simulink model "eovsa_corr_300mhz"  (R2012b)
settings: Solver=VariableStepDiscrete  SolverMode=SingleTasking  StartTime=0.0  StopTime=5000  RelTol=1e-3
undefined symbols (not defined in the file or in its folder): A, B, gcbh, PCIN, sfp, xlBlockLoadCallback, xlipgetpartsetting
libraries: xbsIndex_r4 x5996, casper_library_misc x52, simulink x33, dspsigops x24, xps_library x15, casper_library_delays x2
(part 5 of 65)

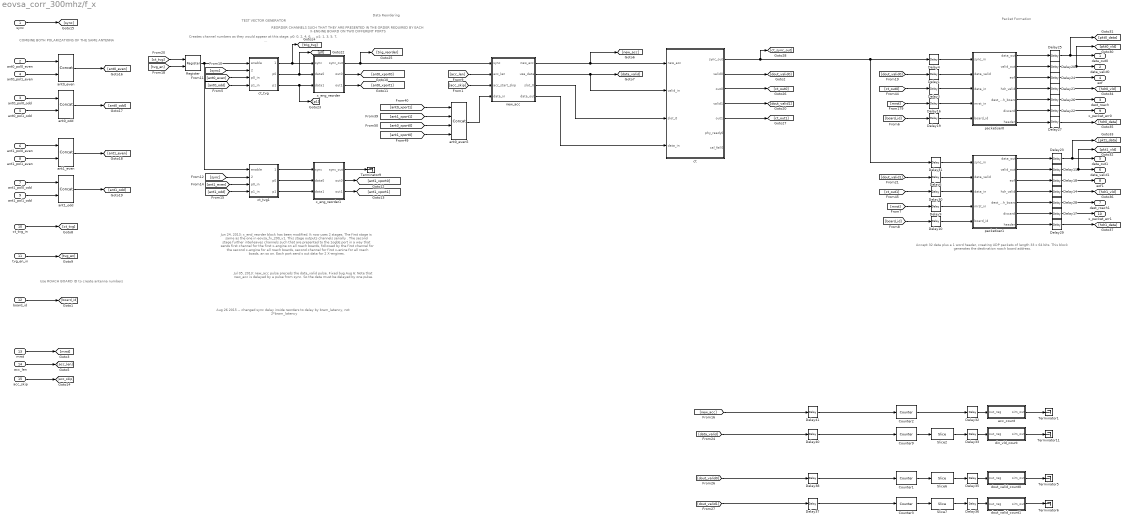
== system eovsa_corr_300mhz/f_x ==
  note: Aug 26 2015 -- changed sync delay inside reorders to delay by bram_latency, not 2*bram_latency
  note: Accept 32 data plus a 1 word header,
      | creating UDP packets of length 33 x 64 bits.
      | This block generates the destination roach board address.
  note: Packet Formation
  note: Data Reordering
  note: COMBINE BOTH POLARIZATIONS
      | OF THE SAME ANTENNA
  note: REORDER CHANNELS SUCH THAT
      | THEY ARE PRESENTED IN THE ORDER
      | REQUIRED BY EACH X-ENGINE BOARD
      | ON TWO DIFFERENT PORTS
  note: TEST VECTOR
      | GENERATOR
  note: Creates channel numbers as they
      | would appear at this stage.
      | p0: 0, 2, 4, 6, ...
      | p1: 1, 3, 5, 7, ...
  note: Jun 24, 2013: x_end_reorder block has been modified.
      | It now uses 2 stages. The first stage is same as the one in eovsa_fx_200_v1.
      | This stage outputs channels serially .
      | The second stage further interleaves channels such that are presented to the 1ogbE port in a way that sends first channel for the first x-engine on all roach boards, followed by
      | the first channel for the second x-engine for all roach boards, second channel for first x-enine for all roach boads, an so on. Each port send s out data for 2 X-engines.
  note: Use ROACH BOARD ID to create antenna numbers
  note: Jul 05, 2013: new_acc  pulse preceds the data_valid pulse. Fixed bug
      | Aug 6: Note that new_acc is delayed by a pulse from sync. So the data must be delayed by one pulse.
  sync : Inport
  ant0_pol0_even : Inport  Port=2
  ant0_pol0_odd : Inport  Port=3
  ant0_pol1_even : Inport  Port=4
  ant0_pol1_odd : Inport  Port=5
  ant1_pol0_even : Inport  Port=6
  ant1_pol0_odd : Inport  Port=7
  ant1_pol1_even : Inport  Port=8
  ant1_pol1_odd : Inport  Port=9
  ct_tvg_in : Inport  Port=10
  tvg_en_in : Inport  Port=11
  board_id : Inport  Port=12
  mrst : Inport  Port=13
  acc_len : Inport  Port=14
  acc_skip : Inport  Port=15
  Counter1 : xbsIndex_r4/Counter  cnt_type=Free Running  cnt_to=Inf  operation=Up  start_count=0  cnt_by_val=1  arith_type=Unsigned  n_bits=32+13  bin_pt=0  load_pin=off  rst=off  en=on  explicit_period=off  period=1  dbl_ovrd=off  use_behavioral_HDL=off  implementation=DSP48  block_type=counter
      settings: block_version=11.4
  Counter2 : xbsIndex_r4/Counter  cnt_type=Free Running  cnt_to=Inf  operation=Up  start_count=0  cnt_by_val=1  arith_type=Unsigned  n_bits=32  bin_pt=0  load_pin=off  rst=off  en=on  explicit_period=off  period=1  dbl_ovrd=off  use_behavioral_HDL=off  implementation=DSP48  block_type=counter
      settings: block_version=11.4
  Counter3 : xbsIndex_r4/Counter  cnt_type=Free Running  cnt_to=Inf  operation=Up  start_count=0  cnt_by_val=1  arith_type=Unsigned  n_bits=32+13  bin_pt=0  load_pin=off  rst=off  en=on  explicit_period=off  period=1  dbl_ovrd=off  use_behavioral_HDL=off  implementation=DSP48  block_type=counter
      settings: block_version=11.4
  Counter9 : xbsIndex_r4/Counter  cnt_type=Free Running  cnt_to=Inf  operation=Up  start_count=0  cnt_by_val=1  arith_type=Unsigned  n_bits=46  bin_pt=0  load_pin=off  rst=off  en=on  explicit_period=off  period=1  dbl_ovrd=off  use_behavioral_HDL=off  implementation=DSP48  block_type=counter
      settings: block_version=11.4
  Delay{1,3,6,30,32..33,35..38,40..41} (12 alike) : xbsIndex_r4/Delay  rst=off  infoeditControl=Selection of Reset will increase slice count due to use of real FFs and instead of SRLs  en=off  latency=1  dbl_ovrd=off  reg_retiming=off  block_type=delay
      settings: xl_area=[0, 0, 0, 0, 0, 0, 0]
  Delay{4,9..11,14,16..29,31} (20 alike) : xbsIndex_r4/Delay  rst=off  infoeditControl=Selection of Reset will increase slice count due to use of real FFs and instead of SRLs  en=off  latency=1  dbl_ovrd=off  reg_retiming=on  block_type=delay
      settings: xl_area=[0, 0, 0, 0, 0, 0, 0]
  Register : xbsIndex_r4/Register  init=0  rst=off  en=on  dbl_ovrd=off  block_type=register
      settings: block_version=11.4
  Slice2 : xbsIndex_r4/Slice  nbits=32  boolean_output=off  mode=Upper Bit Location + Width  bit1=0  base1=MSB of Input  bit0=32  base0=LSB of Input  dbl_ovrd=off  block_type=slice
  Slice6 : xbsIndex_r4/Slice  nbits=32  boolean_output=off  mode=Upper Bit Location + Width  bit1=0  base1=MSB of Input  bit0=32  base0=LSB of Input  dbl_ovrd=off  block_type=slice
  Slice7 : xbsIndex_r4/Slice  nbits=32  boolean_output=off  mode=Upper Bit Location + Width  bit1=0  base1=MSB of Input  bit0=32  base0=LSB of Input  dbl_ovrd=off  block_type=slice
  Terminator{1,5..6,9,11} (5 alike) : Terminator
  acc_count : Subsystem  Tag=xps:sw_reg  AncestorBlock=xps_library/software_register  mask(swreg){mode=one value, io_dir=To Processor, io_delay=0, sample_period=1, names=reg, bitwidths=32, arith_types=0, bin_pts=0, sim_port=on, show_format=off}
      mask prompts: io_dir "I/O direction"; io_delay "I/O delay"; sample_period "Sample period"; names "Name:"; bitwidths "Bitwidth:"; arith_types "Type (ufix=0, fix=1, bool=2):"; bin_pts "Binary pt:"; sim_port "Provide sim input/output?"; show_format "Print format string?"
      mask init:
      | swreg_init(gcb)
      settings: AttributesFormatString=1output
      mask TypeOptions mode: one value | fields of equal size | fields of arbitrary size
      mask Callback mode: swreg_cb(gcb);
      mask TypeOptions io_dir: To Processor | From Processor
      mask Callback io_dir:
      | mask_enables = get_param(gcb, 'MaskEnables');
      | mask_names = get_param(gcb, 'MaskNames');
      | if strcmp(get_param(gcb, 'io_dir'), 'To Processor'),
      |     mask_enables{ismember(mask_names, 'sample_period')} = 'off';
      | else
      |     mask_enables{ismember(mask_names, 'sample_period')} = 'on';
      | end
      | set_param(gcb, 'MaskEnables', mask_enables);
      mask Callback bitwidths:
      | swreg_maskcheck(gcb);
      | % blk = gcb;
      | % mode = get_param(blk, 'mode');
      | % current_widths = eval(get_param(blk, 'bitwidths'));
      | % if (strcmp(mode, 'one value') || strcmp(mode, 'fields of equal size')) && (length(current_widths) > 1),
      | %     error('Only one width may be specified for this mode.');
      | % elseif strcmp(mode, 'fields of arbitrary size')
      | %     current_names = textscan(strtrim(strrep(strrep(get_param(blk, 'names'), ']', ''), '[', '')), '%s');
      | %     current_names = current_names{1};
      | %     numios = length(current_names);
      | %     if length(current_widths) ~= numios,
      | %         error('%d field names specified, but %d widths?', numios, length(current_widths));
      | %     end
      | % end
      | % total_width = 0;
      | % for ctr = 1 : length(current_widths),
      | %     total_width = total_width + current_widths(ctr);
      | % end
      | % if total_width > 32,
      | %     error('Total width must be 32 or less, set to %d.', total_width);
      | % end
      mask Callback arith_types:
      | [numios, ~, ~, ~, current_types] = swreg_maskcheck(gcb);
      | % blk = gcb;
      | % mode = get_param(blk, 'mode');
      | % current_types = eval(get_param(blk, 'arith_types'));
      | % numios = length(current_types);
      | % if (strcmp(mode, 'one value') || strcmp(mode, 'fields of equal size')) && (length(current_types) > 1),
      | %     error('Only one type may be specified for this mode.');
      | % elseif strcmp(mode, 'fields of arbitrary size')
      | %     current_names = textscan(strtrim(strrep(strrep(get_param(blk, 'names'), ']', ''), '[', '')), '%s');
      | %     current_names = current_names{1};
      | %     numios = length(current_names);
      | %     if length(current_types) ~= numios,
      | %         error('%d field names specified, but %d types?', numios, length(current_types));
      | %     end
      | % end
      | problem = 0;
      | for ctr = 1 : numios,
      |     t = current_types(ctr);
      |     if (t < 0) || (t > 2),
      |         problem = t;
      |         ctr = numios + 1;
      |     end
      | end
      | if problem ~= 0,
      |     error('Type cannot be %i, must be 0, 1 or 2.', problem);
      | end
      mask Callback bin_pts:
      | swreg_maskcheck(gcb);
      | % blk = gcb;
      | % mode = get_param(blk, 'mode');
      | % current_bins = eval(get_param(blk, 'bin_pts'));
      | % if (strcmp(mode, 'one value') || strcmp(mode, 'fields of equal size')) && (length(current_bins) > 1),
      | %     error('Only one binary pt may be specified for this mode.');
      | % elseif strcmp(mode, 'fields of arbitrary size')
      | %     current_names = textscan(strtrim(strrep(strrep(get_param(blk, 'names'), ']', ''), '[', '')), '%s');
      | %     current_names = current_names{1};
      | %     numios = length(current_names);
      | %     if length(current_bins) ~= numios,
      | %         error('%d field names specified, but %d binary pts?', numios, length(current_bins));
      | %     end
      | % end
  ant0_even : xbsIndex_r4/Concat  num_inputs=2  dbl_ovrd=off  block_type=concat
  ant0_even5 : xbsIndex_r4/Concat  num_inputs=4  dbl_ovrd=off  block_type=concat
  ant0_odd : xbsIndex_r4/Concat  num_inputs=2  dbl_ovrd=off  block_type=concat
  ant1_even : xbsIndex_r4/Concat  num_inputs=2  dbl_ovrd=off  block_type=concat
  ant1_odd : xbsIndex_r4/Concat  num_inputs=2  dbl_ovrd=off  block_type=concat
  ct : Subsystem  mask{freq_chan=fft_size, x_acc_len=9, bram_latency=3, ip_bits=16}
      mask prompts: freq_chan "No. of frequency channels (2 ^ ?)"; x_acc_len "X-eng Accumulation length (2^? samples):"; bram_latency "bram latency"; ip_bits "Input channel bitwidth"
  ct_tvg : Subsystem  mask{num_channels_bits=fft_size, channel_bits=8, ant=0}
      mask prompts: num_channels_bits "Number of channels (2^?):"; channel_bits "Bits per channel:"; ant "Antenna # [0, 15]"
  ct_tvg1 : Subsystem  mask{num_channels_bits=fft_size, channel_bits=8, ant=1}
      mask prompts: num_channels_bits "Number of channels (2^?):"; channel_bits "Bits per channel:"; ant "Antenna # [0, 15]"
  din_vld_count : Subsystem  Tag=xps:sw_reg  AncestorBlock=xps_library/software_register  mask(swreg){mode=one value, io_dir=To Processor, io_delay=0, sample_period=1, names=reg, bitwidths=32, arith_types=0, bin_pts=0, sim_port=on, show_format=off}
      mask prompts: io_dir "I/O direction"; io_delay "I/O delay"; sample_period "Sample period"; names "Name:"; bitwidths "Bitwidth:"; arith_types "Type (ufix=0, fix=1, bool=2):"; bin_pts "Binary pt:"; sim_port "Provide sim input/output?"; show_format "Print format string?"
      mask init:
      | swreg_init(gcb)
      settings: AttributesFormatString=1output
      mask TypeOptions mode: one value | fields of equal size | fields of arbitrary size
      mask Callback mode: swreg_cb(gcb);
      mask TypeOptions io_dir: To Processor | From Processor
      mask Callback io_dir:
      | mask_enables = get_param(gcb, 'MaskEnables');
      | mask_names = get_param(gcb, 'MaskNames');
      | if strcmp(get_param(gcb, 'io_dir'), 'To Processor'),
      |     mask_enables{ismember(mask_names, 'sample_period')} = 'off';
      | else
      |     mask_enables{ismember(mask_names, 'sample_period')} = 'on';
      | end
      | set_param(gcb, 'MaskEnables', mask_enables);
      mask Callback bitwidths:
      | swreg_maskcheck(gcb);
      | % blk = gcb;
      | % mode = get_param(blk, 'mode');
      | % current_widths = eval(get_param(blk, 'bitwidths'));
      | % if (strcmp(mode, 'one value') || strcmp(mode, 'fields of equal size')) && (length(current_widths) > 1),
      | %     error('Only one width may be specified for this mode.');
      | % elseif strcmp(mode, 'fields of arbitrary size')
      | %     current_names = textscan(strtrim(strrep(strrep(get_param(blk, 'names'), ']', ''), '[', '')), '%s');
      | %     current_names = current_names{1};
      | %     numios = length(current_names);
      | %     if length(current_widths) ~= numios,
      | %         error('%d field names specified, but %d widths?', numios, length(current_widths));
      | %     end
      | % end
      | % total_width = 0;
      | % for ctr = 1 : length(current_widths),
      | %     total_width = total_width + current_widths(ctr);
      | % end
      | % if total_width > 32,
      | %     error('Total width must be 32 or less, set to %d.', total_width);
      | % end
      mask Callback arith_types:
      | [numios, ~, ~, ~, current_types] = swreg_maskcheck(gcb);
      | % blk = gcb;
      | % mode = get_param(blk, 'mode');
      | % current_types = eval(get_param(blk, 'arith_types'));
      | % numios = length(current_types);
      | % if (strcmp(mode, 'one value') || strcmp(mode, 'fields of equal size')) && (length(current_types) > 1),
      | %     error('Only one type may be specified for this mode.');
      | % elseif strcmp(mode, 'fields of arbitrary size')
      | %     current_names = textscan(strtrim(strrep(strrep(get_param(blk, 'names'), ']', ''), '[', '')), '%s');
      | %     current_names = current_names{1};
      | %     numios = length(current_names);
      | %     if length(current_types) ~= numios,
      | %         error('%d field names specified, but %d types?', numios, length(current_types));
      | %     end
      | % end
      | problem = 0;
      | for ctr = 1 : numios,
      |     t = current_types(ctr);
      |     if (t < 0) || (t > 2),
      |         problem = t;
      |         ctr = numios + 1;
      |     end
      | end
      | if problem ~= 0,
      |     error('Type cannot be %i, must be 0, 1 or 2.', problem);
      | end
      mask Callback bin_pts:
      | swreg_maskcheck(gcb);
      | % blk = gcb;
      | % mode = get_param(blk, 'mode');
      | % current_bins = eval(get_param(blk, 'bin_pts'));
      | % if (strcmp(mode, 'one value') || strcmp(mode, 'fields of equal size')) && (length(current_bins) > 1),
      | %     error('Only one binary pt may be specified for this mode.');
      | % elseif strcmp(mode, 'fields of arbitrary size')
      | %     current_names = textscan(strtrim(strrep(strrep(get_param(blk, 'names'), ']', ''), '[', '')), '%s');
      | %     current_names = current_names{1};
      | %     numios = length(current_names);
      | %     if length(current_bins) ~= numios,
      | %         error('%d field names specified, but %d binary pts?', numios, length(current_bins));
      | %     end
      | % end
  dout_valid_count0 : Subsystem  Tag=xps:sw_reg  AncestorBlock=xps_library/software_register  mask(swreg){mode=one value, io_dir=To Processor, io_delay=0, sample_period=1, names=reg, bitwidths=32, arith_types=0, bin_pts=0, sim_port=on, show_format=off}
      mask prompts: io_dir "I/O direction"; io_delay "I/O delay"; sample_period "Sample period"; names "Name:"; bitwidths "Bitwidth:"; arith_types "Type (ufix=0, fix=1, bool=2):"; bin_pts "Binary pt:"; sim_port "Provide sim input/output?"; show_format "Print format string?"
      mask init:
      | swreg_init(gcb)
      settings: AttributesFormatString=1output
      mask TypeOptions mode: one value | fields of equal size | fields of arbitrary size
      mask Callback mode: swreg_cb(gcb);
      mask TypeOptions io_dir: To Processor | From Processor
      mask Callback io_dir:
      | mask_enables = get_param(gcb, 'MaskEnables');
      | mask_names = get_param(gcb, 'MaskNames');
      | if strcmp(get_param(gcb, 'io_dir'), 'To Processor'),
      |     mask_enables{ismember(mask_names, 'sample_period')} = 'off';
      | else
      |     mask_enables{ismember(mask_names, 'sample_period')} = 'on';
      | end
      | set_param(gcb, 'MaskEnables', mask_enables);
      mask Callback bitwidths:
      | swreg_maskcheck(gcb);
      | % blk = gcb;
      | % mode = get_param(blk, 'mode');
      | % current_widths = eval(get_param(blk, 'bitwidths'));
      | % if (strcmp(mode, 'one value') || strcmp(mode, 'fields of equal size')) && (length(current_widths) > 1),
      | %     error('Only one width may be specified for this mode.');
      | % elseif strcmp(mode, 'fields of arbitrary size')
      | %     current_names = textscan(strtrim(strrep(strrep(get_param(blk, 'names'), ']', ''), '[', '')), '%s');
      | %     current_names = current_names{1};
      | %     numios = length(current_names);
      | %     if length(current_widths) ~= numios,
      | %         error('%d field names specified, but %d widths?', numios, length(current_widths));
      | %     end
      | % end
      | % total_width = 0;
      | % for ctr = 1 : length(current_widths),
      | %     total_width = total_width + current_widths(ctr);
      | % end
      | % if total_width > 32,
      | %     error('Total width must be 32 or less, set to %d.', total_width);
      | % end
      mask Callback arith_types:
      | [numios, ~, ~, ~, current_types] = swreg_maskcheck(gcb);
      | % blk = gcb;
      | % mode = get_param(blk, 'mode');
      | % current_types = eval(get_param(blk, 'arith_types'));
      | % numios = length(current_types);
      | % if (strcmp(mode, 'one value') || strcmp(mode, 'fields of equal size')) && (length(current_types) > 1),
      | %     error('Only one type may be specified for this mode.');
      | % elseif strcmp(mode, 'fields of arbitrary size')
      | %     current_names = textscan(strtrim(strrep(strrep(get_param(blk, 'names'), ']', ''), '[', '')), '%s');
      | %     current_names = current_names{1};
      | %     numios = length(current_names);
      | %     if length(current_types) ~= numios,
      | %         error('%d field names specified, but %d types?', numios, length(current_types));
      | %     end
      | % end
      | problem = 0;
      | for ctr = 1 : numios,
      |     t = current_types(ctr);
      |     if (t < 0) || (t > 2),
      |         problem = t;
      |         ctr = numios + 1;
      |     end
      | end
      | if problem ~= 0,
      |     error('Type cannot be %i, must be 0, 1 or 2.', problem);
      | end
      mask Callback bin_pts:
      | swreg_maskcheck(gcb);
      | % blk = gcb;
      | % mode = get_param(blk, 'mode');
      | % current_bins = eval(get_param(blk, 'bin_pts'));
      | % if (strcmp(mode, 'one value') || strcmp(mode, 'fields of equal size')) && (length(current_bins) > 1),
      | %     error('Only one binary pt may be specified for this mode.');
      | % elseif strcmp(mode, 'fields of arbitrary size')
      | %     current_names = textscan(strtrim(strrep(strrep(get_param(blk, 'names'), ']', ''), '[', '')), '%s');
      | %     current_names = current_names{1};
      | %     numios = length(current_names);
      | %     if length(current_bins) ~= numios,
      | %         error('%d field names specified, but %d binary pts?', numios, length(current_bins));
      | %     end
      | % end
  dout_valid_count1 : Subsystem  Tag=xps:sw_reg  AncestorBlock=xps_library/software_register  mask(swreg){mode=one value, io_dir=To Processor, io_delay=0, sample_period=1, names=reg, bitwidths=32, arith_types=0, bin_pts=0, sim_port=on, show_format=off}
      mask prompts: io_dir "I/O direction"; io_delay "I/O delay"; sample_period "Sample period"; names "Name:"; bitwidths "Bitwidth:"; arith_types "Type (ufix=0, fix=1, bool=2):"; bin_pts "Binary pt:"; sim_port "Provide sim input/output?"; show_format "Print format string?"
      mask init:
      | swreg_init(gcb)
      settings: AttributesFormatString=1output
      mask TypeOptions mode: one value | fields of equal size | fields of arbitrary size
      mask Callback mode: swreg_cb(gcb);
      mask TypeOptions io_dir: To Processor | From Processor
      mask Callback io_dir:
      | mask_enables = get_param(gcb, 'MaskEnables');
      | mask_names = get_param(gcb, 'MaskNames');
      | if strcmp(get_param(gcb, 'io_dir'), 'To Processor'),
      |     mask_enables{ismember(mask_names, 'sample_period')} = 'off';
      | else
      |     mask_enables{ismember(mask_names, 'sample_period')} = 'on';
      | end
      | set_param(gcb, 'MaskEnables', mask_enables);
      mask Callback bitwidths:
      | swreg_maskcheck(gcb);
      | % blk = gcb;
      | % mode = get_param(blk, 'mode');
      | % current_widths = eval(get_param(blk, 'bitwidths'));
      | % if (strcmp(mode, 'one value') || strcmp(mode, 'fields of equal size')) && (length(current_widths) > 1),
      | %     error('Only one width may be specified for this mode.');
      | % elseif strcmp(mode, 'fields of arbitrary size')
      | %     current_names = textscan(strtrim(strrep(strrep(get_param(blk, 'names'), ']', ''), '[', '')), '%s');
      | %     current_names = current_names{1};
      | %     numios = length(current_names);
      | %     if length(current_widths) ~= numios,
      | %         error('%d field names specified, but %d widths?', numios, length(current_widths));
      | %     end
      | % end
      | % total_width = 0;
      | % for ctr = 1 : length(current_widths),
      | %     total_width = total_width + current_widths(ctr);
      | % end
      | % if total_width > 32,
      | %     error('Total width must be 32 or less, set to %d.', total_width);
      | % end
      mask Callback arith_types:
      | [numios, ~, ~, ~, current_types] = swreg_maskcheck(gcb);
      | % blk = gcb;
      | % mode = get_param(blk, 'mode');
      | % current_types = eval(get_param(blk, 'arith_types'));
      | % numios = length(current_types);
      | % if (strcmp(mode, 'one value') || strcmp(mode, 'fields of equal size')) && (length(current_types) > 1),
      | %     error('Only one type may be specified for this mode.');
      | % elseif strcmp(mode, 'fields of arbitrary size')
      | %     current_names = textscan(strtrim(strrep(strrep(get_param(blk, 'names'), ']', ''), '[', '')), '%s');
      | %     current_names = current_names{1};
      | %     numios = length(current_names);
      | %     if length(current_types) ~= numios,
      | %         error('%d field names specified, but %d types?', numios, length(current_types));
      | %     end
      | % end
      | problem = 0;
      | for ctr = 1 : numios,
      |     t = current_types(ctr);
      |     if (t < 0) || (t > 2),
      |         problem = t;
      |         ctr = numios + 1;
      |     end
      | end
      | if problem ~= 0,
      |     error('Type cannot be %i, must be 0, 1 or 2.', problem);
      | end
      mask Callback bin_pts:
      | swreg_maskcheck(gcb);
      | % blk = gcb;
      | % mode = get_param(blk, 'mode');
      | % current_bins = eval(get_param(blk, 'bin_pts'));
      | % if (strcmp(mode, 'one value') || strcmp(mode, 'fields of equal size')) && (length(current_bins) > 1),
      | %     error('Only one binary pt may be specified for this mode.');
      | % elseif strcmp(mode, 'fields of arbitrary size')
      | %     current_names = textscan(strtrim(strrep(strrep(get_param(blk, 'names'), ']', ''), '[', '')), '%s');
      | %     current_names = current_names{1};
      | %     numios = length(current_names);
      | %     if length(current_bins) ~= numios,
      | %         error('%d field names specified, but %d binary pts?', numios, length(current_bins));
      | %     end
      | % end
  new_acc : Subsystem
  packetiser0 : Subsystem  mask{payload_bits=9-2+1, n_x_board=2, freq_chan=fft_size, n_boards=3, gbe_port=0, n_ant_merge_bits=1}
      mask prompts: payload_bits "Payload length in 64bit words (2^?)"; n_x_board "Number of x-engines per ROACH board (2^?)"; freq_chan "Number of frequencies (2^?)"; n_boards "Number of  ROACH boards (2 ^ ?)"; gbe_port "Port # (0 or 1)"; n_ant_merge_bits "Antennas to coalesce (2^?)"
      mask help: Package 32 bit data into 64 bits and identify data as coming from antenna 0 or 1
      mask init:
      | n_x = n_x_board - 1;
  packetiser1 : Subsystem  mask{payload_bits=9-2+1, n_x_board=2, freq_chan=fft_size, n_boards=3, gbe_port=1, n_ant_merge_bits=1}
      mask prompts: payload_bits "Payload length in 64bit words (2^?)"; n_x_board "Number of x-engines per ROACH board (2^?)"; freq_chan "Number of frequencies (2^?)"; n_boards "Number of  ROACH boards (2 ^ ?)"; gbe_port "Port # (0 or 1)"; n_ant_merge_bits "Antennas to coalesce (2^?)"
      mask help: Package 32 bit data into 64 bits and identify data as coming from antenna 0 or 1
      mask init:
      | n_x = n_x_board - 1;
  x_eng_reorder : Subsystem  mask{freq_chan=fft_size, num_data_bits=16, bram_latency=3, n_boards=3, n_x_board=2}
      mask prompts: freq_chan "Number of Frequency Channels (2 ^ ?)"; num_data_bits "Incomin data width in bits"; bram_latency "BRAM Latency"; n_boards "Number of ROACH boards (2 ^ ?)"; n_x_board "Number of X-engines per ROACH board (2 ^ ?)"
      mask help:
      | Reorders channels for transmission to X-engines in two stages.
      |
      | In the first stage, total of P channels on both inputs (P/2 on each input)
      | are reordered as follows:
      |
      | Input data0 has channels: 0, 2, 4, ..., P-2.
      | Input data1 has channels: 1, 3, 5, ..., P-1.
      | Then,
      | Output out0 has channels: 0, 1, 2, ..., P/2 -1.
      | Output out1 has channels: P/2, P/2 + 1, ..., P-1.
      |
      | Here P = 2 ^ (N - B),
      | where 2 ^ N = no. of total frequency channels
      | and 2 ^ B = total number of ROACH boards
      |
      | In the second stage, the channels on the each output are reordered in a way
      | that when presented to the 10 GbE port, they appear in the following order:
      | First channel to the first X-engine connected to the receiving 10gbE port of all ROACH boards.
      | First channel to the second X-engine connected to the receiving 10GbE port of all ROACH boards.
      | and so on.
      mask init:
      | n_x = n_x_board - 1;
  x_eng_reorder1 : Subsystem  mask{freq_chan=fft_size, num_data_bits=16, bram_latency=3, n_boards=3, n_x_board=2}
      mask prompts: freq_chan "Number of Frequency Channels (2 ^ ?)"; num_data_bits "Incomin data width in bits"; bram_latency "BRAM Latency"; n_boards "Number of ROACH boards (2 ^ ?)"; n_x_board "Number of X-engines per ROACH board (2 ^ ?)"
      mask help:
      | Reorders channels for transmission to X-engines in two stages.
      |
      | In the first stage, total of P channels on both inputs (P/2 on each input)
      | are reordered as follows:
      |
      | Input data0 has channels: 0, 2, 4, ..., P-2.
      | Input data1 has channels: 1, 3, 5, ..., P-1.
      | Then,
      | Output out0 has channels: 0, 1, 2, ..., P/2 -1.
      | Output out1 has channels: P/2, P/2 + 1, ..., P-1.
      |
      | Here P = 2 ^ (N - B),
      | where 2 ^ N = no. of total frequency channels
      | and 2 ^ B = total number of ROACH boards
      |
      | In the second stage, the channels on the each output are reordered in a way
      | that when presented to the 10 GbE port, they appear in the following order:
      | First channel to the first X-engine connected to the receiving 10gbE port of all ROACH boards.
      | First channel to the second X-engine connected to the receiving 10GbE port of all ROACH boards.
      | and so on.
      mask init:
      | n_x = n_x_board - 1;
  data_out0 : Outport
  data_valid0 : Outport  Port=2
  dest_roach : Outport  Port=3
  eof : Outport  Port=4
  data_out1 : Outport  Port=5
  data_valid1 : Outport  Port=6
  dest_roach1 : Outport  Port=7
  eof1 : Outport  Port=8
  x_packet_err0 : Outport  Port=9
  x_packet_err1 : Outport  Port=10
  wires:
  [ct_tvg] -> Register/1
  [tvg_en] -> Register/2
  Register/1 -> ct_tvg/1(enable), ct_tvg1/1(enable)
  ct_tvg_in/1 -> [ct_tvg]
  tvg_en_in/1 -> [tvg_en]
  board_id/1 -> [board_id]
  mrst/1 -> [mrst]
  ant0_pol0_even/1 -> ant0_even/1
  ant0_pol1_even/1 -> ant0_even/2
  ant0_pol0_odd/1 -> ant0_odd/1
  ant0_pol1_odd/1 -> ant0_odd/2
  ct_tvg/1(sync_out) -> [trig_tvg], x_eng_reorder/1(sync)
  acc_len/1 -> [acc_len]
  [acc_len] -> new_acc/2(acc_len)
  ct_tvg/2(p0) -> [p0], x_eng_reorder/2(data0)
  acc_skip/1 -> [acc_skip]
  [acc_skip] -> new_acc/3(acc_start_skip)
  ct/1(sync_out) -> [ct_sync_out], Delay4/1, Delay31/1
  ct/3(out0) -> [ct_out0]
  ant1_pol0_even/1 -> ant1_even/1
  ant1_pol1_even/1 -> ant1_even/2
  ant1_pol0_odd/1 -> ant1_odd/1
  ant1_pol1_odd/1 -> ant1_odd/2
  sync/1 -> [sync]
  ant0_even/1 -> [ant0_even]
  ant0_odd/1 -> [ant0_odd]
  ant1_even/1 -> [ant1_even]
  ant1_odd/1 -> [ant1_odd]
  [sync] -> ct_tvg/2(sync_in)
  [ant0_even] -> ct_tvg/3(p0_in)
  [ant0_odd] -> ct_tvg/4(p1_in)
  [sync] -> ct_tvg1/2(sync_in)
  [ant1_even] -> ct_tvg1/3(p0_in)
  [ant1_odd] -> ct_tvg1/4(p1_in)
  acc_count/1(sim_out) -> Terminator1/1
  Counter2/1 -> Delay32/1
  dout_valid_count0/1(sim_out) -> Terminator5/1
  Counter1/1 -> Slice6/1
  dout_valid_count1/1(sim_out) -> Terminator6/1
  ct/2(valid0) -> [dout_valid0]
  ct/4(valid1) -> [dout_valid1]
  ct/5(out1) -> [ct_out1]
  Counter9/1 -> Slice2/1
  din_vld_count/1(sim_out) -> Terminator11/1
  ct_tvg/3(p1) -> x_eng_reorder/3(data1), [p1]
  [ant0_xport1] -> ant0_even5/1
  [ant1_xport1] -> ant0_even5/2
  [ant0_xport0] -> ant0_even5/3
  [ant1_xport0] -> ant0_even5/4
  ant0_even5/1 -> new_acc/4(data_in)
  [dout_valid0] -> Delay1/1
  [ct_out0] -> Delay3/1
  [mrst] -> Delay16/1
  [board_id] -> Delay19/1
  Delay4/1 -> packetiser0/1(sync_in)
  Delay1/1 -> packetiser0/2(data_valid)
  Delay3/1 -> packetiser0/3(data_in)
  Delay16/1 -> packetiser0/4(mrst_in)
  Delay19/1 -> packetiser0/5(board_id)
  packetiser0/1(data_out) -> Delay25/1
  packetiser0/2(valid_out) -> Delay20/1
  packetiser0/3(eof) -> Delay24/1
  packetiser0/4(hdr_valid) -> Delay21/1
  packetiser0/7(header) -> Delay27/1
  packetiser0/5(dest_roach_board) -> Delay26/1
  packetiser0/6(discard) -> Delay22/1
  Delay25/1 -> data_out0/1, [pkt0_data]
  Delay20/1 -> data_valid0/1, [pkt0_vld]
  Delay26/1 -> dest_roach/1
  Delay24/1 -> eof/1
  Delay22/1 -> x_packet_err0/1
  Delay21/1 -> [hdr0_vld]
  Delay27/1 -> [hdr0_data]
  [dout_valid1] -> Delay6/1
  [ct_out1] -> Delay30/1
  [mrst] -> Delay9/1
  [board_id] -> Delay10/1
  Delay31/1 -> packetiser1/1(sync_in)
  Delay6/1 -> packetiser1/2(data_valid)
  Delay30/1 -> packetiser1/3(data_in)
  Delay9/1 -> packetiser1/4(mrst_in)
  Delay10/1 -> packetiser1/5(board_id)
  packetiser1/1(data_out) -> Delay23/1
  packetiser1/2(valid_out) -> Delay11/1
  packetiser1/3(eof) -> Delay18/1
  packetiser1/4(hdr_valid) -> Delay14/1
  packetiser1/7(header) -> Delay29/1
  packetiser1/5(dest_roach_board) -> Delay28/1
  packetiser1/6(discard) -> Delay17/1
  Delay23/1 -> [pkt1_data], data_out1/1
  Delay11/1 -> [pkt1_vld], data_valid1/1
  Delay28/1 -> dest_roach1/1
  Delay18/1 -> eof1/1
  Delay17/1 -> x_packet_err1/1
  Delay14/1 -> [hdr1_vld]
  Delay29/1 -> [hdr1_data]
  new_acc/1(new_acc) -> [new_acc], ct/1(new_acc)
  new_acc/2(use_data) -> [data_valid], ct/2(valid_in)
  new_acc/3(slot_0) -> ct/3(slot_0)
  new_acc/4(data_out) -> ct/4(data_in)
  Slice6/1 -> Delay35/1
  Counter3/1 -> Slice7/1
  Slice7/1 -> Delay36/1
  Slice2/1 -> Delay33/1
  Delay32/1 -> acc_count/1(out_reg)
  Delay33/1 -> din_vld_count/1(out_reg)
  Delay35/1 -> dout_valid_count0/1(out_reg)
  Delay36/1 -> dout_valid_count1/1(out_reg)
  Delay37/1 -> Counter3/1
  Delay38/1 -> Counter1/1
  Delay40/1 -> Counter9/1
  Delay41/1 -> Counter2/1
  [dout_valid0] -> Delay38/1
  [dout_valid1] -> Delay37/1
  [new_acc] -> Delay41/1
  [data_valid] -> Delay40/1
  x_eng_reorder/1(sync_out) -> [trig_reorder], new_acc/1(sync)
  x_eng_reorder/2(out0) -> [ant0_xport0]
  x_eng_reorder/3(out1) -> [ant0_xport1]
  ct_tvg1/2(p0) -> x_eng_reorder1/2(data0)
  ct_tvg1/3(p1) -> x_eng_reorder1/3(data1)
  ct_tvg1/1(sync_out) -> x_eng_reorder1/1(sync)
  x_eng_reorder1/1(sync_out) -> Terminator9/1
  x_eng_reorder1/2(out0) -> [ant1_xport0]
  x_eng_reorder1/3(out1) -> [ant1_xport1]

== system eovsa_corr_300mhz/ip0 ==
  addr : Inport
  data_in : Inport  Port=2
  we : Inport  Port=3
  calc_add : Subsystem  mask{data_width=32, addr_width=10, sample_rate=sample_rate}
      mask prompts: data_width "data width"; addr_width "address width"; sample_rate "sample rate"
  convert_addr : xbsIndex_r4/Convert  gui_display_data_type=Fixed-point  arith_type=Unsigned  n_bits=addr_width  bin_pt=0  float_type=Single  exp_bits=8  fraction_bits=24  quantization=Truncate  overflow=Wrap  en=off  latency=0  dbl_ovrd=off  pipeline=off  block_type=convert
      settings: xl_area=[0, 0, 0, 0, 0, 0, 0]
  convert_din1 : xbsIndex_r4/Convert  gui_display_data_type=Fixed-point  arith_type=Unsigned  n_bits=32  bin_pt=0  float_type=Single  exp_bits=8  fraction_bits=24  quantization=Truncate  overflow=Wrap  en=off  latency=0  dbl_ovrd=off  pipeline=off  block_type=convert
      settings: xl_area=[0, 0, 0, 0, 0, 0, 0]
  convert_we : xbsIndex_r4/Convert  gui_display_data_type=Fixed-point  arith_type=Unsigned  n_bits=1  bin_pt=0  float_type=Single  exp_bits=8  fraction_bits=24  quantization=Truncate  overflow=Wrap  en=off  latency=0  dbl_ovrd=off  pipeline=off  block_type=convert
      settings: xl_area=[0, 0, 0, 0, 0, 0, 0]
  eovsa_corr_300mhz_ip0_addr : xbsIndex_r4/Gateway Out  inherit_from_input=off  hdl_port=on  timing_constraint=None  locs_specified=off  LOCs={'A5','B9','A9','C1','A3','G6','E9','A6','A7','A8','B8','B1','B3','D9','B5','B4','B6','C2'}  UseAsDAC=off  DACChannel='1'  block_type=gatewayout
      settings: infoedit="Gateway out block.  Converts Xilinx fixed point inputs into ouputs of type Simulink integer, double, or fixed point.<P><P>Hardware notes:  In hardware these blocks become top level output ports or are discarded, depending on how they are configured."  xl_area=[0, 0, 0, 0, 0, 0, 0]  sginterface={'Nallatech'=>{'xdspkit'=>{'non_memory_mapped_port'=>'uprev_Shared_BRAM_addr'}},'Xilinx'=>{'jtaghwcosim'=>{'non_memory_mapped_port'=>'uprev_Shared_BRAM_addr'},'xdspkit'=>{'non_memory_mapped_port'=>'uprev_Shared_BRAM_addr'}}}
  eovsa_corr_300mhz_ip0_data_in : xbsIndex_r4/Gateway Out  inherit_from_input=off  hdl_port=on  timing_constraint=None  locs_specified=off  LOCs={'B21','B22','A22','B23','B19','C19','A20','A21','A23','B24','A24','A25','E18','D18','C18','B18'}  UseAsDAC=off  DACChannel='1'  block_type=gatewayout
      settings: infoedit="Gateway out block.  Converts Xilinx fixed point inputs into ouputs of type Simulink integer, double, or fixed point.<P><P>Hardware notes:  In hardware these blocks become top level output ports or are discarded, depending on how they are configured."  xl_area=[0, 0, 0, 0, 0, 0, 0]  sginterface={'Nallatech'=>{'xdspkit'=>{'non_memory_mapped_port'=>'uprev_Shared_BRAM_data_in'}},'Xilinx'=>{'jtaghwcosim'=>{'non_memory_mapped_port'=>'uprev_Shared_BRAM_data_in'},'xdspkit'=>{'non_memory_mapped_port'=>'uprev_Shared_BRAM_data_in'}}}
  eovsa_corr_300mhz_ip0_data_out : xbsIndex_r4/Gateway In  gui_display_data_type=Fixed-point  arith_type=Unsigned  n_bits=32  bin_pt=0  preci_type=Single  exp_width=8  frac_width=24  quantization=Truncate  overflow=Wrap  period=sample_rate  dbl_ovrd=off  timing_constraint=None  locs_specified=off  LOCs={}  UseAsADC=off  ADCChannel='1'  inherit_from_input=off  hdl_port=on  block_type=gatewayin
      settings: xl_area=[0, 0, 0, 0, 0, 0, 0]
  eovsa_corr_300mhz_ip0_we : xbsIndex_r4/Gateway Out  inherit_from_input=off  hdl_port=on  timing_constraint=None  locs_specified=off  LOCs={'A14'}  UseAsDAC=off  DACChannel='1'  block_type=gatewayout
      settings: infoedit="Gateway out block.  Converts Xilinx fixed point inputs into ouputs of type Simulink integer, double, or fixed point.<P><P>Hardware notes:  In hardware these blocks become top level output ports or are discarded, depending on how they are configured."  xl_area=[0, 0, 0, 0, 0, 0, 0]
  mem : Subsystem
  munge_in : Subsystem  AncestorBlock=casper_library_flow_control/munge  mask(munge){divisions=1, div_size=32, order=[0], arith_type_out=Unsigned, bin_pt_out=0}
      mask prompts: divisions "Number of divisions"; div_size "Division size (bits)"; order "Division packing order"; arith_type_out "Output arithmetic type"; bin_pt_out "Output binary point"
      mask help: Splits an input bus into the specified number of divisions and then recombines them in the order specified (most significant division = 0,least = number divisions-1)
      mask init:
      | munge_init(gcb, ...
      |     'divisions', divisions, ...
      |     'div_size', div_size, ...
      |     'order', order, ...
      |     'arith_type_out', arith_type_out, ...
      |     'bin_pt_out', bin_pt_out);
      settings: AttributesFormatString=|
      | split:32
      | join:0
      | Unsigned [32,0]
      mask TypeOptions arith_type_out: Unsigned | Signed  (2's comp) | Floating-point
  munge_out : Subsystem  AncestorBlock=casper_library_flow_control/munge  mask(munge){divisions=1, div_size=32, order=[0], arith_type_out=Unsigned, bin_pt_out=0}
      mask prompts: divisions "Number of divisions"; div_size "Division size (bits)"; order "Division packing order"; arith_type_out "Output arithmetic type"; bin_pt_out "Output binary point"
      mask help: Splits an input bus into the specified number of divisions and then recombines them in the order specified (most significant division = 0,least = number divisions-1)
      mask init:
      | munge_init(gcb, ...
      |     'divisions', divisions, ...
      |     'div_size', div_size, ...
      |     'order', order, ...
      |     'arith_type_out', arith_type_out, ...
      |     'bin_pt_out', bin_pt_out);
      settings: AttributesFormatString=|
      | split:32
      | join:0
      | Unsigned [32,0]
      mask TypeOptions arith_type_out: Unsigned | Signed  (2's comp) | Floating-point
  data_out : Outport
  wires:
  convert_addr/1 -> eovsa_corr_300mhz_ip0_addr/1
  convert_din1/1 -> eovsa_corr_300mhz_ip0_data_in/1
  data_in/1 -> munge_in/1(din)
  calc_add/1(out) -> convert_addr/1
  eovsa_corr_300mhz_ip0_we/1 -> mem/3(In3)
  eovsa_corr_300mhz_ip0_data_in/1 -> mem/2(In2)
  eovsa_corr_300mhz_ip0_addr/1 -> mem/1(In1)
  convert_we/1 -> eovsa_corr_300mhz_ip0_we/1
  eovsa_corr_300mhz_ip0_data_out/1 -> munge_out/1(din)
  mem/1(Out1) -> eovsa_corr_300mhz_ip0_data_out/1
  addr/1 -> calc_add/1(in)
  we/1 -> convert_we/1
  munge_out/1(dout) -> data_out/1
  munge_in/1(dout) -> convert_din1/1

== system eovsa_corr_300mhz/ip1 ==
  addr : Inport
  data_in : Inport  Port=2
  we : Inport  Port=3
  calc_add : Subsystem  mask{data_width=32, addr_width=10, sample_rate=sample_rate}
      mask prompts: data_width "data width"; addr_width "address width"; sample_rate "sample rate"
  convert_addr : xbsIndex_r4/Convert  gui_display_data_type=Fixed-point  arith_type=Unsigned  n_bits=addr_width  bin_pt=0  float_type=Single  exp_bits=8  fraction_bits=24  quantization=Truncate  overflow=Wrap  en=off  latency=0  dbl_ovrd=off  pipeline=off  block_type=convert
      settings: xl_area=[0, 0, 0, 0, 0, 0, 0]
  convert_din1 : xbsIndex_r4/Convert  gui_display_data_type=Fixed-point  arith_type=Unsigned  n_bits=32  bin_pt=0  float_type=Single  exp_bits=8  fraction_bits=24  quantization=Truncate  overflow=Wrap  en=off  latency=0  dbl_ovrd=off  pipeline=off  block_type=convert
      settings: xl_area=[0, 0, 0, 0, 0, 0, 0]
  convert_we : xbsIndex_r4/Convert  gui_display_data_type=Fixed-point  arith_type=Unsigned  n_bits=1  bin_pt=0  float_type=Single  exp_bits=8  fraction_bits=24  quantization=Truncate  overflow=Wrap  en=off  latency=0  dbl_ovrd=off  pipeline=off  block_type=convert
      settings: xl_area=[0, 0, 0, 0, 0, 0, 0]
  eovsa_corr_300mhz_ip1_addr : xbsIndex_r4/Gateway Out  inherit_from_input=off  hdl_port=on  timing_constraint=None  locs_specified=off  LOCs={'A5','B9','A9','C1','A3','G6','E9','A6','A7','A8','B8','B1','B3','D9','B5','B4','B6','C2'}  UseAsDAC=off  DACChannel='1'  block_type=gatewayout
      settings: infoedit="Gateway out block.  Converts Xilinx fixed point inputs into ouputs of type Simulink integer, double, or fixed point.<P><P>Hardware notes:  In hardware these blocks become top level output ports or are discarded, depending on how they are configured."  xl_area=[0, 0, 0, 0, 0, 0, 0]  sginterface={'Nallatech'=>{'xdspkit'=>{'non_memory_mapped_port'=>'uprev_Shared_BRAM_addr'}},'Xilinx'=>{'jtaghwcosim'=>{'non_memory_mapped_port'=>'uprev_Shared_BRAM_addr'},'xdspkit'=>{'non_memory_mapped_port'=>'uprev_Shared_BRAM_addr'}}}
  eovsa_corr_300mhz_ip1_data_in : xbsIndex_r4/Gateway Out  inherit_from_input=off  hdl_port=on  timing_constraint=None  locs_specified=off  LOCs={'B21','B22','A22','B23','B19','C19','A20','A21','A23','B24','A24','A25','E18','D18','C18','B18'}  UseAsDAC=off  DACChannel='1'  block_type=gatewayout
      settings: infoedit="Gateway out block.  Converts Xilinx fixed point inputs into ouputs of type Simulink integer, double, or fixed point.<P><P>Hardware notes:  In hardware these blocks become top level output ports or are discarded, depending on how they are configured."  xl_area=[0, 0, 0, 0, 0, 0, 0]  sginterface={'Nallatech'=>{'xdspkit'=>{'non_memory_mapped_port'=>'uprev_Shared_BRAM_data_in'}},'Xilinx'=>{'jtaghwcosim'=>{'non_memory_mapped_port'=>'uprev_Shared_BRAM_data_in'},'xdspkit'=>{'non_memory_mapped_port'=>'uprev_Shared_BRAM_data_in'}}}
  eovsa_corr_300mhz_ip1_data_out : xbsIndex_r4/Gateway In  gui_display_data_type=Fixed-point  arith_type=Unsigned  n_bits=32  bin_pt=0  preci_type=Single  exp_width=8  frac_width=24  quantization=Truncate  overflow=Wrap  period=sample_rate  dbl_ovrd=off  timing_constraint=None  locs_specified=off  LOCs={}  UseAsADC=off  ADCChannel='1'  inherit_from_input=off  hdl_port=on  block_type=gatewayin
      settings: xl_area=[0, 0, 0, 0, 0, 0, 0]
  eovsa_corr_300mhz_ip1_we : xbsIndex_r4/Gateway Out  inherit_from_input=off  hdl_port=on  timing_constraint=None  locs_specified=off  LOCs={'A14'}  UseAsDAC=off  DACChannel='1'  block_type=gatewayout
      settings: infoedit="Gateway out block.  Converts Xilinx fixed point inputs into ouputs of type Simulink integer, double, or fixed point.<P><P>Hardware notes:  In hardware these blocks become top level output ports or are discarded, depending on how they are configured."  xl_area=[0, 0, 0, 0, 0, 0, 0]
  mem : Subsystem
  munge_in : Subsystem  AncestorBlock=casper_library_flow_control/munge  mask(munge){divisions=1, div_size=32, order=[0], arith_type_out=Unsigned, bin_pt_out=0}
      mask prompts: divisions "Number of divisions"; div_size "Division size (bits)"; order "Division packing order"; arith_type_out "Output arithmetic type"; bin_pt_out "Output binary point"
      mask help: Splits an input bus into the specified number of divisions and then recombines them in the order specified (most significant division = 0,least = number divisions-1)
      mask init:
      | munge_init(gcb, ...
      |     'divisions', divisions, ...
      |     'div_size', div_size, ...
      |     'order', order, ...
      |     'arith_type_out', arith_type_out, ...
      |     'bin_pt_out', bin_pt_out);
      settings: AttributesFormatString=|
      | split:32
      | join:0
      | Unsigned [32,0]
      mask TypeOptions arith_type_out: Unsigned | Signed  (2's comp) | Floating-point
  munge_out : Subsystem  AncestorBlock=casper_library_flow_control/munge  mask(munge){divisions=1, div_size=32, order=[0], arith_type_out=Unsigned, bin_pt_out=0}
      mask prompts: divisions "Number of divisions"; div_size "Division size (bits)"; order "Division packing order"; arith_type_out "Output arithmetic type"; bin_pt_out "Output binary point"
      mask help: Splits an input bus into the specified number of divisions and then recombines them in the order specified (most significant division = 0,least = number divisions-1)
      mask init:
      | munge_init(gcb, ...
      |     'divisions', divisions, ...
      |     'div_size', div_size, ...
      |     'order', order, ...
      |     'arith_type_out', arith_type_out, ...
      |     'bin_pt_out', bin_pt_out);
      settings: AttributesFormatString=|
      | split:32
      | join:0
      | Unsigned [32,0]
      mask TypeOptions arith_type_out: Unsigned | Signed  (2's comp) | Floating-point
  data_out : Outport
  wires:
  munge_in/1(dout) -> convert_din1/1
  munge_out/1(dout) -> data_out/1
  we/1 -> convert_we/1
  addr/1 -> calc_add/1(in)
  mem/1(Out1) -> eovsa_corr_300mhz_ip1_data_out/1
  eovsa_corr_300mhz_ip1_data_out/1 -> munge_out/1(din)
  convert_we/1 -> eovsa_corr_300mhz_ip1_we/1
  eovsa_corr_300mhz_ip1_addr/1 -> mem/1(In1)
  eovsa_corr_300mhz_ip1_data_in/1 -> mem/2(In2)
  eovsa_corr_300mhz_ip1_we/1 -> mem/3(In3)
  calc_add/1(out) -> convert_addr/1
  data_in/1 -> munge_in/1(din)
  convert_din1/1 -> eovsa_corr_300mhz_ip1_data_in/1
  convert_addr/1 -> eovsa_corr_300mhz_ip1_addr/1

== system eovsa_corr_300mhz/masker1 ==
  sync : Inport
  din : Inport  Port=2
  vld : Inport  Port=3
  mcnt : Inport  Port=4
  Delay1 : xbsIndex_r4/Delay  rst=off  infoeditControl=Selection of Reset will increase slice count due to use of real FFs and instead of SRLs  en=off  latency=1  dbl_ovrd=off  reg_retiming=on  block_type=delay
      settings: block_version=11.4
  Delay33 : xbsIndex_r4/Delay  rst=off  infoeditControl=Selection of Reset will increase slice count due to use of real FFs and instead of SRLs  en=off  latency=1  dbl_ovrd=off  reg_retiming=on  block_type=delay
      settings: block_version=11.4
  Inverter1 : xbsIndex_r4/Inverter  en=off  latency=0  dbl_ovrd=off  block_type=inv
  Inverter2 : xbsIndex_r4/Inverter  en=off  latency=0  dbl_ovrd=off  block_type=inv
  Register : xbsIndex_r4/Register  init=0  rst=on  en=off  dbl_ovrd=off  block_type=register
  Register1 : xbsIndex_r4/Register  init=0  rst=on  en=off  dbl_ovrd=off  block_type=register
  sync_out : Outport
  dout : Outport  Port=2
  vld_out : Outport  Port=3
  mcnt_out : Outport  Port=4
  wires:
  Delay1/1 -> sync_out/1
  sync/1 -> Delay1/1
  Delay33/1 -> vld_out/1
  mcnt/1 -> Register1/1
  Register1/1 -> mcnt_out/1
  vld/1 -> Inverter1/1, Inverter2/1, Delay33/1
  Register/1 -> dout/1
  din/1 -> Register/1
  Inverter1/1 -> Register/2
  Inverter2/1 -> Register1/2

== system eovsa_corr_300mhz/masker2 ==
  sync : Inport
  din : Inport  Port=2
  vld : Inport  Port=3
  mcnt : Inport  Port=4
  Delay1 : xbsIndex_r4/Delay  rst=off  infoeditControl=Selection of Reset will increase slice count due to use of real FFs and instead of SRLs  en=off  latency=1  dbl_ovrd=off  reg_retiming=on  block_type=delay
      settings: block_version=11.4
  Delay33 : xbsIndex_r4/Delay  rst=off  infoeditControl=Selection of Reset will increase slice count due to use of real FFs and instead of SRLs  en=off  latency=1  dbl_ovrd=off  reg_retiming=on  block_type=delay
      settings: block_version=11.4
  Inverter1 : xbsIndex_r4/Inverter  en=off  latency=0  dbl_ovrd=off  block_type=inv
  Inverter2 : xbsIndex_r4/Inverter  en=off  latency=0  dbl_ovrd=off  block_type=inv
  Register : xbsIndex_r4/Register  init=0  rst=on  en=off  dbl_ovrd=off  block_type=register
  Register1 : xbsIndex_r4/Register  init=0  rst=on  en=off  dbl_ovrd=off  block_type=register
  sync_out : Outport
  dout : Outport  Port=2
  vld_out : Outport  Port=3
  mcnt_out : Outport  Port=4
  wires:
  Inverter2/1 -> Register1/2
  Inverter1/1 -> Register/2
  din/1 -> Register/1
  Register/1 -> dout/1
  vld/1 -> Delay33/1, Inverter2/1, Inverter1/1
  Register1/1 -> mcnt_out/1
  mcnt/1 -> Register1/1
  Delay33/1 -> vld_out/1
  sync/1 -> Delay1/1
  Delay1/1 -> sync_out/1
